simulink model "ovi"  (R2017a)
settings: Solver=VariableStepAuto  StartTime=0.0  StopTime=10.0  RelTol=1e-3
settings Model: Creator=Vlad Petrenciuc  LastModifiedBy=Vlad Petrenciuc

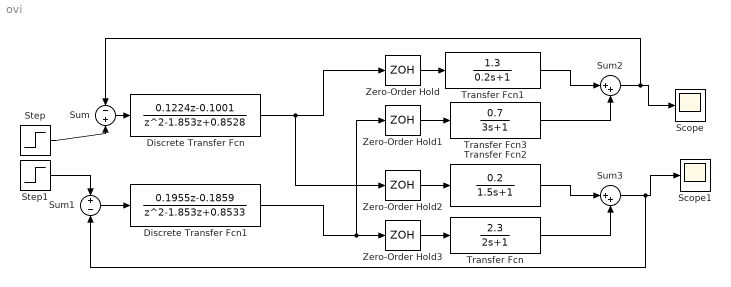
== system ovi ==
  Discrete Transfer Fcn : DiscreteTransferFcn  Numerator=[0.1224 -0.1001]  Denominator=[1 -1.853 0.8528]  SampleTime=0.1
  Discrete Transfer Fcn1 : DiscreteTransferFcn  Numerator=[0.1955 -0.1859]  Denominator=[1 -1.853 0.8533]
  Scope : Scope
  Scope1 : Scope
  Step : Step  After=0  SampleTime=0
  Step1 : Step  SampleTime=0
  Sum : Sum  Inputs=-+
  Sum1 : Sum  Inputs=+-
  Sum2 : Sum  Inputs=|++
  Sum3 : Sum  Inputs=|++
  Transfer Fcn : TransferFcn  Numerator=[2.3]  Denominator=[2 1]
  Transfer Fcn1 : TransferFcn  Numerator=[1.3]  Denominator=[0.2 1]
  Transfer Fcn2 : TransferFcn  Numerator=[0.2]  Denominator=[1.5 1]
  Transfer Fcn3 : TransferFcn  Numerator=[0.7]  Denominator=[3 1]
  Zero-Order Hold{,1..3} (4 alike) : ZeroOrderHold  SampleTime=0.1
  wires:
  Sum/1 -> Discrete Transfer Fcn/1
  Zero-Order Hold/1 -> Transfer Fcn1/1
  Zero-Order Hold1/1 -> Transfer Fcn3/1
  Zero-Order Hold2/1 -> Transfer Fcn2/1
  Zero-Order Hold3/1 -> Transfer Fcn/1
  Sum1/1 -> Discrete Transfer Fcn1/1
  Step/1 -> Sum/2
  Step1/1 -> Sum1/1
  Sum2/1 -> Sum/1, Scope/1
  Transfer Fcn3/1 -> Sum2/2
  Transfer Fcn1/1 -> Sum2/1
  Transfer Fcn/1 -> Sum3/2
  Transfer Fcn2/1 -> Sum3/1
  Sum3/1 -> Sum1/2, Scope1/1
  Discrete Transfer Fcn/1 -> Zero-Order Hold2/1, Zero-Order Hold/1
  Discrete Transfer Fcn1/1 -> Zero-Order Hold1/1, Zero-Order Hold3/1
